simulink model "magNoise"  (R2013a)
settings: Solver=ode45  StartTime=0.0  StopTime=t  RelTol=1e-3
values from neighbouring files (symbols this model uses):
  sampleTime = mydata.sampleTime    [runtracklsq.m]    (also in workspace.mat = 0.01)
libraries: simulink x12
settings Model: Creator=User  LastModifiedBy=User

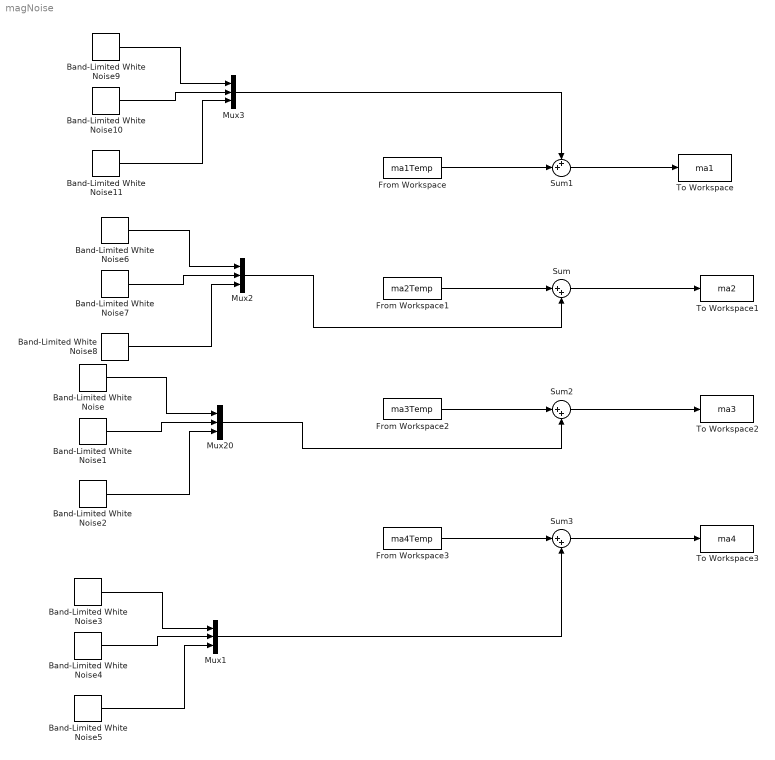
== system magNoise ==
  Band-Limited White Noise{,1..11} (12 alike) : simulink/Sources/Band-Limited White Noise  Cov=[0.01*0.8671E-5*0.5]  Ts=sampleTime  seed=[23341]
  From Workspace : FromWorkspace  VariableName=ma1Temp  SampleTime=sampleTime
  From Workspace1 : FromWorkspace  VariableName=ma2Temp  SampleTime=sampleTime
  From Workspace2 : FromWorkspace  VariableName=ma3Temp  SampleTime=sampleTime
  From Workspace3 : FromWorkspace  VariableName=ma4Temp  SampleTime=sampleTime
  Mux{1..3,20} (4 alike) : Mux  Inputs=3
  Sum : Sum  Inputs=|++
  Sum1 : Sum  Inputs=++|
  Sum2 : Sum  Inputs=|++
  Sum3 : Sum  Inputs=|++
  To Workspace : ToWorkspace  VariableName=ma1  SampleTime=sampleTime  SaveFormat=Structure With Time
  To Workspace1 : ToWorkspace  VariableName=ma2  SampleTime=sampleTime  SaveFormat=Structure With Time
  To Workspace2 : ToWorkspace  VariableName=ma3  SampleTime=sampleTime  SaveFormat=Structure With Time
  To Workspace3 : ToWorkspace  VariableName=ma4  SampleTime=sampleTime  SaveFormat=Structure With Time
  wires:
  From Workspace/1 -> Sum1/2
  From Workspace1/1 -> Sum/1
  Sum1/1 -> To Workspace/1
  Sum/1 -> To Workspace1/1
  From Workspace2/1 -> Sum2/1
  Sum2/1 -> To Workspace2/1
  From Workspace3/1 -> Sum3/1
  Sum3/1 -> To Workspace3/1
  Band-Limited White Noise/1 -> Mux20/1
  Band-Limited White Noise1/1 -> Mux20/2
  Band-Limited White Noise2/1 -> Mux20/3
  Band-Limited White Noise3/1 -> Mux1/1
  Band-Limited White Noise4/1 -> Mux1/2
  Band-Limited White Noise5/1 -> Mux1/3
  Band-Limited White Noise6/1 -> Mux2/1
  Band-Limited White Noise7/1 -> Mux2/2
  Band-Limited White Noise8/1 -> Mux2/3
  Band-Limited White Noise9/1 -> Mux3/1
  Band-Limited White Noise10/1 -> Mux3/2
  Band-Limited White Noise11/1 -> Mux3/3
  Mux3/1 -> Sum1/1
  Mux2/1 -> Sum/2
  Mux20/1 -> Sum2/2
  Mux1/1 -> Sum3/2
